simulink model "gm_Lab2_farrow_impl"  (R2022a)
settings: Solver=VariableStepAuto  StartTime=0.0  StopTime=0.3  RelTol=1e-3
libraries: simulink x1
settings Model: Creator=jeldon  LastModifiedBy=duong
settings SolverCC: AlgebraicLoopSolver=TrustRegion
settings OptimizationCC: BlockReduction=off  ConditionallyExecuteInputs=off  DefaultParameterBehavior=Inlined
settings DebuggingCC: AlgebraicLoopMsg=error  InheritedTsInSrcMsg=none  UnconnectedInputMsg=warning  UnconnectedOutputMsg=warning  UnconnectedLineMsg=warning  SFMachineParentedDataDiag=warning
settings HardwareCC: ProdBitPerPointer=32  ProdBitPerSizeT=32  ProdBitPerPtrDiffT=32  ProdLargestAtomicFloat=None  ProdIntDivRoundTo=Undefined  ProdEndianess=Unspecified  ProdWordSize=32  ProdHWDeviceType=ASIC/FPGA->ASIC/FPGA  TargetBitPerPointer=64  TargetBitPerSizeT=64  TargetBitPerPtrDiffT=64  TargetLongLongMode=on  TargetIntDivRoundTo=Zero  TargetEndianess=LittleEndian  TargetWordSize=64  TargetHWDeviceType=Custom Processor->MATLAB Host Computer  ProdEqTarget=off

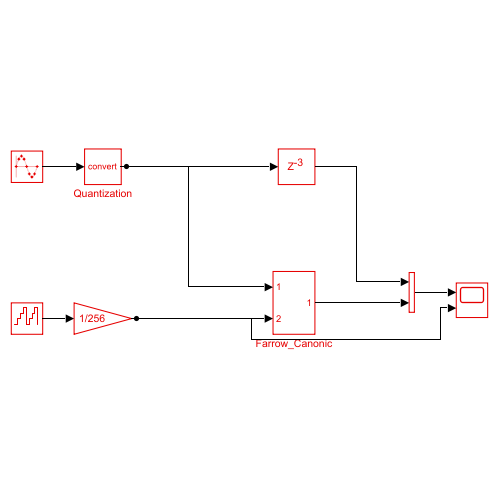
[thumbnail: Simulink's stored preview of the top-level diagram]
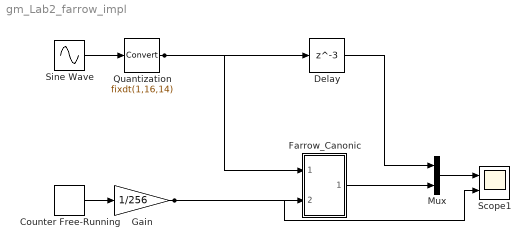
== system gm_Lab2_farrow_impl ==
  Counter Free-Running : simulink/Sources/Counter Free-Running  NumBits=10  tsamp=-1
  Delay : Delay  DelayLength=3  InitialCondition=0
  Farrow_Canonic : Subsystem
  Gain : Gain  Gain=1/256  OutDataTypeStr=fixdt(0,12,8)
  Mux : Mux  Inputs=2
  Quantization : DataTypeConversion  OutDataTypeStr=fixdt(1,16,14)  RndMeth=Convergent  SaturateOnIntegerOverflow=off
  Scope1 : Scope  NumInputPorts=2
  Sine Wave : Sin  SineType=Sample based  Samples=32  SampleTime=.0001
  wires:
  Quantization/1 -> Delay/1, Farrow_Canonic/1(In1)
  Farrow_Canonic/1(Out1) -> Mux/2
  Mux/1 -> Scope1/1
  Counter Free-Running/1 -> Gain/1
  Gain/1 -> Farrow_Canonic/2(In2), Scope1/2
  Delay/1 -> Mux/1
  Sine Wave/1 -> Quantization/1

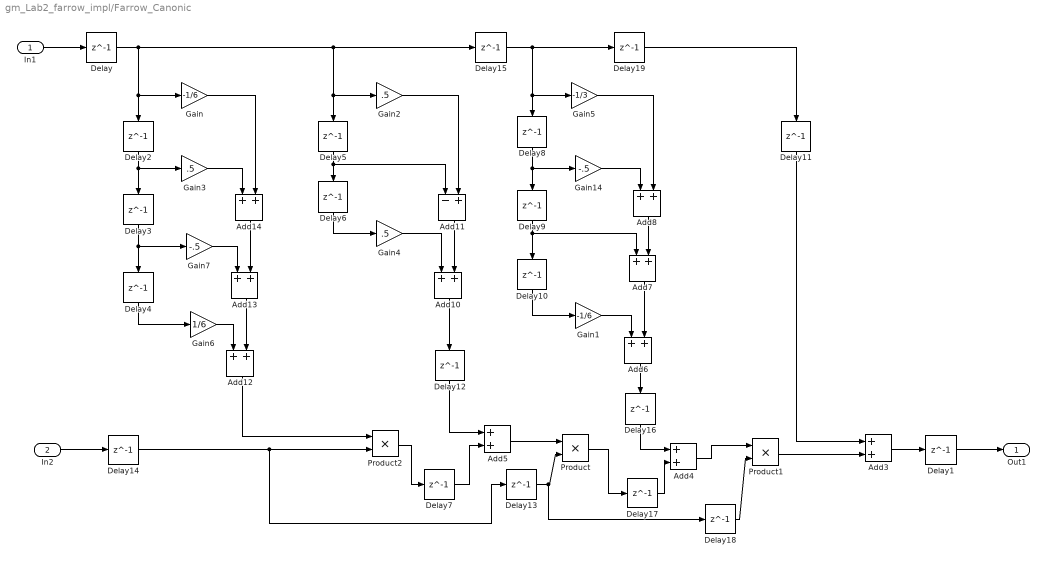
== system gm_Lab2_farrow_impl/Farrow_Canonic ==
  In1 : Inport
  In2 : Inport  Port=2
  Add{7..8,10,13..14} (5 alike) : Sum
  Add11 : Sum  Inputs=-+
  Add12 : Sum  OutDataTypeStr=fixdt(1,24,20)
  Add3 : Sum  OutDataTypeStr=fixdt(1,16,14)  RndMeth=Round
  Add4 : Sum  OutDataTypeStr=Inherit: Same as first input
  Add5 : Sum  OutDataTypeStr=fixdt(1,24,20)  RndMeth=Round
  Add6 : Sum  OutDataTypeStr=fixdt(1,24,20)
  Delay{,1..19} (20 alike) : Delay  DelayLength=1  InitialCondition=0
  Gain : Gain  Gain=-1/6  OutDataTypeStr=fixdt(1,24,20)  RndMeth=Round
  Gain1 : Gain  Gain=-1/6  OutDataTypeStr=fixdt(1,24,20)  RndMeth=Round
  Gain14 : Gain  Gain=-.5  RndMeth=Round  OutDataTypeStr=Inherit: Same as input
  Gain2 : Gain  Gain=.5  RndMeth=Round  OutDataTypeStr=Inherit: Same as input
  Gain3 : Gain  Gain=.5  RndMeth=Round  OutDataTypeStr=Inherit: Same as input
  Gain4 : Gain  Gain=.5  RndMeth=Round  OutDataTypeStr=Inherit: Same as input
  Gain5 : Gain  Gain=-1/3  OutDataTypeStr=fixdt(1,24,20)  RndMeth=Round
  Gain6 : Gain  Gain=1/6  OutDataTypeStr=fixdt(1,24,20)  RndMeth=Round
  Gain7 : Gain  Gain=-.5  RndMeth=Round  OutDataTypeStr=Inherit: Same as input
  Product : Product  RndMeth=Round  OutDataTypeStr=Inherit: Same as first input
  Product1 : Product
  Product2 : Product  RndMeth=Round  OutDataTypeStr=Inherit: Same as first input
  Out1 : Outport
  wires:
  Delay19/1 -> Delay11/1
  Delay18/1 -> Product1/2
  Add6/1 -> Delay16/1
  Delay16/1 -> Add4/1
  Delay17/1 -> Add4/2
  Product/1 -> Delay17/1
  Delay15/1 -> Delay19/1, Delay8/1, Gain5/1
  Delay13/1 -> Product/2, Delay18/1
  Delay12/1 -> Add5/1
  Add10/1 -> Delay12/1
  Delay7/1 -> Add5/2
  Product2/1 -> Delay7/1
  Delay9/1 -> Delay10/1, Add7/1
  Gain14/1 -> Add8/1
  Add4/1 -> Product1/1
  Gain4/1 -> Add10/1
  Product1/1 -> Add3/2
  Gain1/1 -> Add6/1
  Add8/1 -> Add7/2
  Add13/1 -> Add12/2
  Add12/1 -> Product2/1
  Add7/1 -> Add6/2
  Add5/1 -> Product/1
  Delay5/1 -> Delay6/1, Add11/1
  Gain6/1 -> Add12/1
  Gain5/1 -> Add8/2
  Delay10/1 -> Gain1/1
  Delay8/1 -> Delay9/1, Gain14/1
  Delay4/1 -> Gain6/1
  Gain2/1 -> Add11/2
  Delay6/1 -> Gain4/1
  Add3/1 -> Delay1/1
  In2/1 -> Delay14/1
  Delay11/1 -> Add3/1
  In1/1 -> Delay/1
  Gain/1 -> Add14/2
  Delay/1 -> Delay2/1, Gain/1, Delay15/1, Gain2/1, Delay5/1
  Delay14/1 -> Product2/2, Delay13/1
  Gain3/1 -> Add14/1
  Delay1/1 -> Out1/1
  Delay2/1 -> Delay3/1, Gain3/1
  Gain7/1 -> Add13/1
  Delay3/1 -> Delay4/1, Gain7/1
  Add14/1 -> Add13/2
  Add11/1 -> Add10/2
